simulink model "Target_Control_System"  (R2021b)
settings: Solver=FixedStepDiscrete  StartTime=0.0  StopTime=5  RelTol=1e-3
PreLoadFcn:
  | RTWConfigurationCB('preloadfcn', bdroot);
PostLoadFcn:
  | load('configuration/data_struct.mat');
  | load('configuration/fluxMaps_propMotor.mat');
  | load('configuration/parameterInit_PROP.mat');
  | load('configuration/parameterInit_PUMP.mat');
  | load('configuration/parameterInit_PITCH.mat');
  | load('configuration/parameterInit_TILT.mat');
  | %load('configuration/base_workspace_signal_definition.mat');
  | %load('resolvedatastores_to_baseworkspace_for_faster_simulation.mat');
model workspace (MAT data in the model file):
  SIMULATION_OPTIONS : Simulink.Parameter (value not decoded)
  TARGET_CODE_GEN : Simulink.Parameter (value not decoded)
  TCS_SAMPLE_FREQ_HZ : Simulink.Parameter (value not decoded)
symbols that are objects in the model workspace (value not decoded): TARGET_CODE_GEN, TCS_SAMPLE_FREQ_HZ
undefined symbols (not defined in the file): A_DQ_REF_LPF_INIT__PITCH, A_DQ_REF_LPF_INIT__PROP, A_DQ_REF_LPF_INIT__PUMP, A_DQ_REF_LPF_INIT__TILT, A_OBSERVER_CONFIDENCE_INIT__PITCH, A_OBSERVER_CONFIDENCE_INIT__PROP, A_OBSERVER_CONFIDENCE_INIT__PUMP, A_OBSERVER_CONFIDENCE_INIT__TILT, ACTUATOR_MAX_ANGLE_TRIP__PITCH, ACTUATOR_MIN_ANGLE_TRIP__PITCH, ACTUATOR_POS_SENSOR_INV_DIRECTION__PITCH, ACTUATOR_POS_SENSOR_INV_DIRECTION__TILT, ACTUATOR_POS_SENSOR_OFFSET__PITCH, ACTUATOR_POS_SENSOR_OFFSET__TILT, ADC_scaler1_baseaddr_TILT, ADC_SCALER_FLOAT_TO_FIXPOINT_EXPANSION, ANGLE_ELEC_FROM_SENSOR_OFFSET_INIT__PITCH, ANGLE_ELEC_FROM_SENSOR_OFFSET_INIT__PROP, ANGLE_ELEC_FROM_SENSOR_OFFSET_INIT__PUMP, ANGLE_ELEC_FROM_SENSOR_OFFSET_INIT__TILT, AUTO_CLEAR_FAULTS_ENABLED__PITCH, AUTO_CLEAR_FAULTS_ENABLED__PROP, AUTO_CLEAR_FAULTS_ENABLED__PUMP, AUTO_CLEAR_FAULTS_ENABLED__TILT, AUTO_CLEAR_FAULTS_WAIT_TICKS__PITCH, AUTO_CLEAR_FAULTS_WAIT_TICKS__PROP, AUTO_CLEAR_FAULTS_WAIT_TICKS__PUMP, AUTO_CLEAR_FAULTS_WAIT_TICKS__TILT, AUTO_I_ZERO_IDLE_TICKS__PITCH, AUTO_I_ZERO_IDLE_TICKS__PROP, AUTO_I_ZERO_IDLE_TICKS__PUMP, AUTO_I_ZERO_IDLE_TICKS__TILT, AUTO_I_ZERO_OFFSET_IDC_THRESHOLD__PITCH, AUTO_I_ZERO_OFFSET_IDC_THRESHOLD__PROP, AUTO_I_ZERO_OFFSET_IDC_THRESHOLD__PUMP, AUTO_I_ZERO_OFFSET_IDC_THRESHOLD__TILT, AUTO_I_ZERO_OFFSET_IPH_THRESHOLD__PITCH, AUTO_I_ZERO_OFFSET_IPH_THRESHOLD__PROP, AUTO_I_ZERO_OFFSET_IPH_THRESHOLD__PUMP, AUTO_I_ZERO_OFFSET_IPH_THRESHOLD__TILT, AUTO_SENSORLESS_SWITCHOVER_DISABLE_OMEGA, AUTO_SENSORLESS_SWITCHOVER_ENABLE_OMEGA, AUTO_SENSORLESS_SWITCHOVER_MIN_CONFIDENCE, AUXILIARY_PROTECTION_UNIT_BASEADDR__TILT, blanking_max_error_omega_INIT_PITCH, blanking_max_error_omega_INIT_TILT, blanking_max_error_position_INIT_PITCH, blanking_max_error_position_INIT_TILT, BRUTE_START_I_Q_REF_RAMP_SPEED__PITCH, BRUTE_START_I_Q_REF_RAMP_SPEED__PROP, BRUTE_START_I_Q_REF_RAMP_SPEED__PUMP, BRUTE_START_I_Q_REF_RAMP_SPEED__TILT, CONTROL_LOOP_DT_INIT__PITCH, CONTROL_LOOP_DT_INIT__PROP, CONTROL_LOOP_DT_INIT__PUMP, CONTROL_LOOP_DT_INIT__TILT, CORRECTION_FILTER_SCALE__PITCH, CORRECTION_FILTER_SCALE__PROP, CORRECTION_FILTER_SCALE__PUMP, CORRECTION_FILTER_SCALE__TILT ... (+458)
libraries: simulink x178, Reusables_Lib x24
(part 39 of 47)

== system Target_Control_System/Target_Control_System/MainLoop/tiltMotor_mainLoop/mainTask_tilt/motorTaskMainFastStep(&oTilt)/Mechanical System - Tilt/processSensors(&oPitch)/Output (actuator) side sensor ==
  note: // Ensure the angle is within -pi/2 to pi*1.5 (no loop needed, assuming 'fActuatorSensorOffsetAngle_' is within -pi to pi)
      |    // The reason for this 'skewed' wrap around angle: the tilt sensor on the linkage style tilts moves between 0 and 200 deg,
      |    // so it'd be mighty convenient if it doesn't wrap around at 180 deg. The flaps have a similar situation.
      |    // For pivot style tilt and VP, the sensor moves between -15 deg and 100 deg at most, so the the shifted wrapping point is a non-issue.
  Add1 : Sum
  Add2 : Sum
  Constant20 : Constant  Value=pi  OutDataTypeStr=single  SampleTime=-1
  Constant21 : Constant  Value=2*pi  OutDataTypeStr=single  SampleTime=-1
  Constant23 : Constant  Value=pi  OutDataTypeStr=single  SampleTime=-1
  Constant24 : Constant  Value=2*pi  OutDataTypeStr=single  SampleTime=-1
  Data Store Read1 : DataStoreRead  DataStoreName=oTilt  DataStoreElements=oTilt.oMot_.oState_.oPosSensor_.iActuatorSensorInverseDirection_  IndexOptions=Index vector (dialog)  Indices=1  OutputSizes=1
  Data Store Read2 : DataStoreRead  DataStoreName=oTilt  DataStoreElements=oTilt.oMot_.oIn_.oAdcData_.fOutputEncoderFloat_  IndexOptions=Index vector (dialog)  Indices=1  OutputSizes=1
  Data Store Read3 : DataStoreRead  DataStoreName=oTilt  DataStoreElements=oTilt.oMot_.oState_.oPosSensor_.fActuatorSensorOffsetAngle_  IndexOptions=Index vector (dialog)  Indices=1  OutputSizes=1
  Data Store Write1 : DataStoreWrite  DataStoreName=oTilt  DataStoreElements=oTilt.oMot_.oState_.oPosSensor_.fActuatorAngleFromSensor_  IndexOptions=Index vector (dialog)  Indices=1  OutputSizes=1
  Subtract3 : Sum  Inputs=+-
  Subtract4 : Sum  Inputs=+-
  Subtract8 : Sum  Inputs=-+
  Switch13 : Switch  Criteria=u2 > Threshold
  Switch15 : Switch  Criteria=u2 > Threshold  Threshold=1.5*pi
  Switch5 : Switch  Threshold=-pi/2.0
  wires:
  Subtract8/1 -> Switch15/1
  Constant24/1 -> Add2/2
  Add1/1 -> Subtract8/2, Add2/1, Switch5/2, Switch5/1, Switch15/2
  Data Store Read3/1 -> Add1/1
  Add2/1 -> Switch5/3
  Subtract4/1 -> Switch13/3
  Data Store Read2/1 -> Subtract3/2, Subtract4/1
  Data Store Read1/1 -> Switch13/2
  Subtract3/1 -> Switch13/1
  Constant21/1 -> Subtract8/1
  Switch5/1 -> Switch15/3
  Constant23/1 -> Subtract3/1
  Constant20/1 -> Subtract4/2
  Switch15/1 -> Data Store Write1/1
  Switch13/1 -> Add1/2

== system Target_Control_System/Target_Control_System/MainLoop/tiltMotor_mainLoop/mainTask_tilt/motorTaskMainFastStep(&oTilt)/Motor Acceleration - Tilt/First filter stage/softwareIirFilterStep() ==
  newInput : Inport
  afConstantsB0 : Inport  Port=2
  afConstantsB1 : Inport  Port=3
  afConstantsB2 : Inport  Port=4
  afConstantsA0 : Inport  Port=5
  afConstantsA1 : Inport  Port=6
  afConstantsA2 : Inport  Port=7
  afPreviousInputs0 : Inport  Port=8
  afPreviousInputs1 : Inport  Port=9
  afPreviousOutputs0 : Inport  Port=10
  afPreviousOutputs1 : Inport  Port=11
  Add : Sum  Inputs=+++--
  Constant : Constant  Value=0  OutDataTypeStr=single  SampleTime=-1
  Constant1 : Constant  Value=0  OutDataTypeStr=single  SampleTime=-1
  Divide{,1..5} (6 alike) : Product  Inputs=**
  IsInf : RelationalOperator  Operator=isInf  OutDataTypeStr=boolean  RndMeth=Simplest
  IsInf1 : RelationalOperator  Operator=isInf  OutDataTypeStr=boolean  RndMeth=Simplest
  IsNaN : RelationalOperator  Operator=isNaN  OutDataTypeStr=boolean  RndMeth=Simplest
  IsNaN1 : RelationalOperator  Operator=isNaN  OutDataTypeStr=boolean  RndMeth=Simplest
  Switch{,1..3} (4 alike) : Switch  Criteria=u2 > Threshold
  *afPreviousInputs1 : Outport
  *afPreviousInputs0 : Outport  Port=2
  *afPreviousOutputs1 : Outport  Port=3
  *afPreviousOutputs0 : Outport  Port=4
  fFilterOutput : Outport  Port=5
  wires:
  Switch3/1 -> Divide5/1, *afPreviousOutputs0/1
  IsInf1/1 -> Switch3/2
  IsNaN1/1 -> Switch2/2
  Constant1/1 -> Switch2/1, Switch3/1
  Switch2/1 -> IsInf1/1, Switch3/3
  Add/1 -> IsNaN1/1, Switch2/3  "fOutput"
  Switch1/1 -> Divide/1, *afPreviousInputs0/1
  Switch/1 -> IsInf/1, Switch1/3
  IsInf/1 -> Switch1/2
  Constant/1 -> Switch/1, Switch1/1
  IsNaN/1 -> Switch/2
  Divide5/1 -> fFilterOutput/1
  afConstantsA0/1 -> Divide5/2
  afPreviousOutputs1/1 -> Divide4/1
  afConstantsA2/1 -> Divide4/2
  afPreviousOutputs0/1 -> Divide3/1, *afPreviousOutputs1/1
  afConstantsA1/1 -> Divide3/2
  afPreviousInputs1/1 -> Divide2/1
  afConstantsB2/1 -> Divide2/2
  Divide4/1 -> Add/5
  Divide3/1 -> Add/4
  Divide/1 -> Add/1
  Divide1/1 -> Add/2
  Divide2/1 -> Add/3
  afPreviousInputs0/1 -> Divide1/1, *afPreviousInputs1/1
  afConstantsB1/1 -> Divide1/2
  newInput/1 -> IsNaN/1, Switch/3
  afConstantsB0/1 -> Divide/2

== system Target_Control_System/Target_Control_System/MainLoop/tiltMotor_mainLoop/mainTask_tilt/motorTaskMainFastStep(&oTilt)/Software Overcurrent Protection - Tilt/checkForHwOvercurrents(&oTilt)/gateDriverStatus ==
  note: 1) Add Subsystem or Model blocks as valid variant choices.
      | 2) You cannot connect blocks at this level. At simulation, connectivity is automatically
      | determined, based on the active variant and port name matching.
  DoNotIncludeCustomCode : Subsystem  TreatAsAtomicUnit=on  VariantControl=TARGET_CODE_GEN == 0
  IncludeCustomCode : Subsystem  TreatAsAtomicUnit=on  VariantControl=(default)

== system Target_Control_System/Target_Control_System/Simulation Controls/Simulation Data Store Initialization/setTiltMotorSpecificParameters()/Enabled Subsystem MotorType/Switch Case Action Subsystem MotorType3/softwareIirFilterInitialize()/computeCoefficientsButter() ==
  fCutoffFrequencyHz : Inport  OutDataTypeStr=single
  dSampleFrequencyHz : Inport  Port=2  OutDataTypeStr=single
  Add : Sum  Inputs=+++  OutDataTypeStr=double
  Add1 : Sum  Inputs=-+
  Add2 : Sum  Inputs=+-+  OutDataTypeStr=double
  Constant : Constant  Value=0.0008  OutDataTypeStr=single
  Constant1 : Constant  Value=0.45  OutDataTypeStr=single
  Constant{5,7,9..10} (4 alike) : Constant
  Constant2 : Constant  Value=pi  OutDataTypeStr=double
  Constant3 : Constant  OutDataTypeStr=double
  Constant4 : Constant  Value=sqrt(2)  OutDataTypeStr=double
  Constant6 : Constant  OutDataTypeStr=double
  Constant8 : Constant  Value=2
  Data Type Conversion : DataTypeConversion  OutDataTypeStr=double
  Divide : Product  Inputs=**  OutDataTypeStr=single
  Divide1 : Product  Inputs=**  OutDataTypeStr=single
  Divide{3,5..6,8,10..11} (6 alike) : Product  Inputs=**  OutDataTypeStr=double
  Divide2 : Product  Inputs=*/  OutDataTypeStr=double
  Divide4 : Product  Inputs=*/  OutDataTypeStr=double
  Divide7 : Product  Inputs=*/  OutDataTypeStr=double
  Divide9 : Product  Inputs=***  OutDataTypeStr=double
  Gain : Gain  Gain=2  OutDataTypeStr=double
  Gain1 : Gain  Gain=-1  OutDataTypeStr=double
  Gain2 : Gain  Gain=-1  OutDataTypeStr=double
  Gain3 : Gain  Gain=-1  OutDataTypeStr=double
  Mux : Mux  Inputs=6
  Saturation Dynamic : simulink/Discontinuities/Saturation Dynamic  OutMin=[]  OutMax=[]  OutDataTypeStr=Inherit: Same as second input  OutDataType=fixdt(1, 16)  OutScaling=2^-10  DoSatur=off
  Tan : Trigonometry  Operator=tan
  dpOutArray : Outport
  fFreq3db : Outport  Port=2
  wires:
  Divide/1 -> Saturation Dynamic/3
  Constant1/1 -> Divide1/1
  dSampleFrequencyHz/1 -> Divide/1, Divide2/2, Divide1/2
  Divide1/1 -> Saturation Dynamic/1
  fCutoffFrequencyHz/1 -> Saturation Dynamic/2  "fCutoffFrequencyHz"
  Constant/1 -> Divide/2
  Divide2/1 -> Divide3/1  "dFf"
  Constant2/1 -> Divide3/2
  Divide3/1 -> Tan/1
  Tan/1 -> Divide4/2
  Constant3/1 -> Divide4/1
  Divide4/1 -> [kdIta]
  Constant4/1 -> [kdQ]
  Mux/1 -> dpOutArray/1
  [kdIta] -> Divide6/2, Divide6/1, Divide5/1
  [kdQ] -> Divide5/2
  Divide6/1 -> Add/1
  Divide5/1 -> Add/2
  Constant5/1 -> Add/3
  Constant6/1 -> Divide7/1
  Add/1 -> Divide7/2
  Divide7/1 -> Divide11/1, Divide9/1, [dB2], Gain/1, [dB0]
  Gain/1 -> [dB1]
  [kdIta] -> Divide10/1, Divide8/2, Divide8/1
  Add1/1 -> Divide9/2
  Constant8/1 -> Divide9/3
  Divide9/1 -> [dA1]
  Divide8/1 -> Add2/1, Add1/2
  Constant7/1 -> Add1/1
  [kdQ] -> Divide10/2
  Divide10/1 -> Add2/2
  Constant9/1 -> Add2/3
  Add2/1 -> Gain1/1
  Gain1/1 -> Divide11/2
  Divide11/1 -> [dA2]
  [dB0] -> Mux/1
  [dB1] -> Mux/2
  [dB2] -> Mux/3
  Gain2/1 -> Mux/5
  [dA1] -> Gain2/1
  Gain3/1 -> Mux/6
  [dA2] -> Gain3/1
  Constant10/1 -> Mux/4
  Data Type Conversion/1 -> Divide2/1
  Saturation Dynamic/1 -> fFreq3db/1, Data Type Conversion/1  "fCutoffFrequencyHz"

== system Target_Control_System/Target_Control_System/Simulation Controls/Simulation Data Store Initialization/setupPwm(&oTilt)/setPwmFrequencyApplication()_tilt/setPwmFrequency()_tilt/softwareIirFilterInitialize()/computeCoefficientsButter() ==
  fCutoffFrequencyHz : Inport  OutDataTypeStr=single
  dSampleFrequencyHz : Inport  Port=2  OutDataTypeStr=single
  Add : Sum  Inputs=+++  OutDataTypeStr=double
  Add1 : Sum  Inputs=-+
  Add2 : Sum  Inputs=+-+  OutDataTypeStr=double
  Constant : Constant  Value=0.0008  OutDataTypeStr=single
  Constant1 : Constant  Value=0.45  OutDataTypeStr=single
  Constant{5,7,9..10} (4 alike) : Constant
  Constant2 : Constant  Value=pi  OutDataTypeStr=double
  Constant3 : Constant  OutDataTypeStr=double
  Constant4 : Constant  Value=sqrt(2)  OutDataTypeStr=double
  Constant6 : Constant  OutDataTypeStr=double
  Constant8 : Constant  Value=2
  Data Type Conversion : DataTypeConversion  OutDataTypeStr=double
  Divide : Product  Inputs=**  OutDataTypeStr=single
  Divide1 : Product  Inputs=**  OutDataTypeStr=single
  Divide{3,5..6,8,10..11} (6 alike) : Product  Inputs=**  OutDataTypeStr=double
  Divide2 : Product  Inputs=*/  OutDataTypeStr=double
  Divide4 : Product  Inputs=*/  OutDataTypeStr=double
  Divide7 : Product  Inputs=*/  OutDataTypeStr=double
  Divide9 : Product  Inputs=***  OutDataTypeStr=double
  Gain : Gain  Gain=2  OutDataTypeStr=double
  Gain1 : Gain  Gain=-1  OutDataTypeStr=double
  Gain2 : Gain  Gain=-1  OutDataTypeStr=double
  Gain3 : Gain  Gain=-1  OutDataTypeStr=double
  Mux : Mux  Inputs=6
  Saturation Dynamic : simulink/Discontinuities/Saturation Dynamic  OutMin=[]  OutMax=[]  OutDataTypeStr=Inherit: Same as second input  OutDataType=fixdt(1, 16)  OutScaling=2^-10  DoSatur=off
  Tan : Trigonometry  Operator=tan
  dpOutArray : Outport
  fFreq3db : Outport  Port=2
  wires:
  Saturation Dynamic/1 -> Data Type Conversion/1, fFreq3db/1  "fCutoffFrequencyHz"
  Data Type Conversion/1 -> Divide2/1
  Constant10/1 -> Mux/4
  [dA2] -> Gain3/1
  Gain3/1 -> Mux/6
  [dA1] -> Gain2/1
  Gain2/1 -> Mux/5
  [dB2] -> Mux/3
  [dB1] -> Mux/2
  [dB0] -> Mux/1
  Divide11/1 -> [dA2]
  Gain1/1 -> Divide11/2
  Add2/1 -> Gain1/1
  Constant9/1 -> Add2/3
  Divide10/1 -> Add2/2
  [kdQ] -> Divide10/2
  Constant7/1 -> Add1/1
  Divide8/1 -> Add1/2, Add2/1
  Divide9/1 -> [dA1]
  Constant8/1 -> Divide9/3
  Add1/1 -> Divide9/2
  [kdIta] -> Divide8/1, Divide8/2, Divide10/1
  Gain/1 -> [dB1]
  Divide7/1 -> [dB0], Gain/1, [dB2], Divide9/1, Divide11/1
  Add/1 -> Divide7/2
  Constant6/1 -> Divide7/1
  Constant5/1 -> Add/3
  Divide5/1 -> Add/2
  Divide6/1 -> Add/1
  [kdQ] -> Divide5/2
  [kdIta] -> Divide5/1, Divide6/1, Divide6/2
  Mux/1 -> dpOutArray/1
  Constant4/1 -> [kdQ]
  Divide4/1 -> [kdIta]
  Constant3/1 -> Divide4/1
  Tan/1 -> Divide4/2
  Divide3/1 -> Tan/1
  Constant2/1 -> Divide3/2
  Divide2/1 -> Divide3/1  "dFf"
  Constant/1 -> Divide/2
  fCutoffFrequencyHz/1 -> Saturation Dynamic/2  "fCutoffFrequencyHz"
  Divide1/1 -> Saturation Dynamic/1
  dSampleFrequencyHz/1 -> Divide1/2, Divide2/2, Divide/1
  Constant1/1 -> Divide1/1
  Divide/1 -> Saturation Dynamic/3

== system Target_Control_System/Target_Control_System/Simulation Controls/Simulation Data Store Initialization/setupPwm(&oTilt)/setPwmFrequencyApplication()_tilt/setPwmFrequency()_tilt/softwareIirFilterInitialize()1/computeCoefficientsButter() ==
  fCutoffFrequencyHz : Inport  OutDataTypeStr=single
  dSampleFrequencyHz : Inport  Port=2  OutDataTypeStr=single
  Add : Sum  Inputs=+++  OutDataTypeStr=double
  Add1 : Sum  Inputs=-+
  Add2 : Sum  Inputs=+-+  OutDataTypeStr=double
  Constant : Constant  Value=0.0008  OutDataTypeStr=single
  Constant1 : Constant  Value=0.45  OutDataTypeStr=single
  Constant{5,7,9..10} (4 alike) : Constant
  Constant2 : Constant  Value=pi  OutDataTypeStr=double
  Constant3 : Constant  OutDataTypeStr=double
  Constant4 : Constant  Value=sqrt(2)  OutDataTypeStr=double
  Constant6 : Constant  OutDataTypeStr=double
  Constant8 : Constant  Value=2
  Data Type Conversion : DataTypeConversion  OutDataTypeStr=double
  Divide : Product  Inputs=**  OutDataTypeStr=single
  Divide1 : Product  Inputs=**  OutDataTypeStr=single
  Divide{3,5..6,8,10..11} (6 alike) : Product  Inputs=**  OutDataTypeStr=double
  Divide2 : Product  Inputs=*/  OutDataTypeStr=double
  Divide4 : Product  Inputs=*/  OutDataTypeStr=double
  Divide7 : Product  Inputs=*/  OutDataTypeStr=double
  Divide9 : Product  Inputs=***  OutDataTypeStr=double
  Gain : Gain  Gain=2  OutDataTypeStr=double
  Gain1 : Gain  Gain=-1  OutDataTypeStr=double
  Gain2 : Gain  Gain=-1  OutDataTypeStr=double
  Gain3 : Gain  Gain=-1  OutDataTypeStr=double
  Mux : Mux  Inputs=6
  Saturation Dynamic : simulink/Discontinuities/Saturation Dynamic  OutMin=[]  OutMax=[]  OutDataTypeStr=Inherit: Same as second input  OutDataType=fixdt(1, 16)  OutScaling=2^-10  DoSatur=off
  Tan : Trigonometry  Operator=tan
  dpOutArray : Outport
  fFreq3db : Outport  Port=2
  wires:
  Saturation Dynamic/1 -> Data Type Conversion/1, fFreq3db/1
  Data Type Conversion/1 -> Divide2/1
  Constant10/1 -> Mux/4
  [dA2] -> Gain3/1
  Gain3/1 -> Mux/6
  [dA1] -> Gain2/1
  Gain2/1 -> Mux/5
  [dB2] -> Mux/3
  [dB1] -> Mux/2
  [dB0] -> Mux/1
  Divide11/1 -> [dA2]
  Gain1/1 -> Divide11/2
  Add2/1 -> Gain1/1
  Constant9/1 -> Add2/3
  Divide10/1 -> Add2/2
  [kdQ] -> Divide10/2
  Constant7/1 -> Add1/1
  Divide8/1 -> Add1/2, Add2/1
  Divide9/1 -> [dA1]
  Constant8/1 -> Divide9/3
  Add1/1 -> Divide9/2
  [kdIta] -> Divide8/1, Divide8/2, Divide10/1
  Gain/1 -> [dB1]
  Divide7/1 -> [dB0], Gain/1, [dB2], Divide9/1, Divide11/1
  Add/1 -> Divide7/2
  Constant6/1 -> Divide7/1
  Constant5/1 -> Add/3
  Divide5/1 -> Add/2
  Divide6/1 -> Add/1
  [kdQ] -> Divide5/2
  [kdIta] -> Divide5/1, Divide6/1, Divide6/2
  Mux/1 -> dpOutArray/1
  Constant4/1 -> [kdQ]
  Divide4/1 -> [kdIta]
  Constant3/1 -> Divide4/1
  Tan/1 -> Divide4/2
  Divide3/1 -> Tan/1
  Constant2/1 -> Divide3/2
  Divide2/1 -> Divide3/1  "dFf"
  Constant/1 -> Divide/2
  fCutoffFrequencyHz/1 -> Saturation Dynamic/2  "fCutoffFrequencyHz"
  Divide1/1 -> Saturation Dynamic/1
  dSampleFrequencyHz/1 -> Divide1/2, Divide2/2, Divide/1
  Constant1/1 -> Divide1/1
  Divide/1 -> Saturation Dynamic/3

== system Target_Control_System/Target_Control_System/Simulation Controls/Simulation Data Store Initialization/setupPwm(&oTilt)/setPwmFrequencyApplication()_tilt/setPwmFrequency()_tilt/updateServoObserver()_tilt/softwareIirFilterInitialize() ==
  fFreq3db : Inport
  fFreqSample : Inport  Port=2  OutDataTypeStr=single
  Constant : Constant  OutDataTypeStr=single
  Constant1 : Constant  Value=0  OutDataTypeStr=single
  Data Store Write : DataStoreWrite  DataStoreName=oTilt  DataStoreElements=oTilt.oMot_.oState_.oPosSensor_.oInputSensorSpeedFilter_.afConstantsA_.h0  IndexOptions=Index vector (dialog)  Indices=1  OutputSizes=1
  Data Store Write1 : DataStoreWrite  DataStoreName=oTilt  DataStoreElements=oTilt.oMot_.oState_.oPosSensor_.oInputSensorSpeedFilter_.afConstantsA_.h1  IndexOptions=Index vector (dialog)  Indices=1  OutputSizes=1
  Data Store Write10 : DataStoreWrite  DataStoreName=oTilt  DataStoreElements=oTilt.oMot_.oState_.oPosSensor_.oInputSensorSpeedFilter_.fFilterOutput_  IndexOptions=Index vector (dialog)  Indices=1  OutputSizes=1
  Data Store Write2 : DataStoreWrite  DataStoreName=oTilt  DataStoreElements=oTilt.oMot_.oState_.oPosSensor_.oInputSensorSpeedFilter_.afConstantsA_.h2  IndexOptions=Index vector (dialog)  Indices=1  OutputSizes=1
  Data Store Write3 : DataStoreWrite  DataStoreName=oTilt  DataStoreElements=oTilt.oMot_.oState_.oPosSensor_.oInputSensorSpeedFilter_.afConstantsB_.h2  IndexOptions=Index vector (dialog)  Indices=1  OutputSizes=1
  Data Store Write4 : DataStoreWrite  DataStoreName=oTilt  DataStoreElements=oTilt.oMot_.oState_.oPosSensor_.oInputSensorSpeedFilter_.afConstantsB_.h1  IndexOptions=Index vector (dialog)  Indices=1  OutputSizes=1
  Data Store Write5 : DataStoreWrite  DataStoreName=oTilt  DataStoreElements=oTilt.oMot_.oState_.oPosSensor_.oInputSensorSpeedFilter_.afConstantsB_.h0  IndexOptions=Index vector (dialog)  Indices=1  OutputSizes=1
  Data Store Write6 : DataStoreWrite  DataStoreName=oTilt  DataStoreElements=oTilt.oMot_.oState_.oPosSensor_.oInputSensorSpeedFilter_.afPreviousInputs_.h0  IndexOptions=Index vector (dialog)  Indices=1  OutputSizes=1
  Data Store Write7 : DataStoreWrite  DataStoreName=oTilt  DataStoreElements=oTilt.oMot_.oState_.oPosSensor_.oInputSensorSpeedFilter_.afPreviousInputs_.h1  IndexOptions=Index vector (dialog)  Indices=1  OutputSizes=1
  Data Store Write8 : DataStoreWrite  DataStoreName=oTilt  DataStoreElements=oTilt.oMot_.oState_.oPosSensor_.oInputSensorSpeedFilter_.afPreviousOutputs_.h0  IndexOptions=Index vector (dialog)  Indices=1  OutputSizes=1
  Data Store Write9 : DataStoreWrite  DataStoreName=oTilt  DataStoreElements=oTilt.oMot_.oState_.oPosSensor_.oInputSensorSpeedFilter_.afPreviousOutputs_.h1  IndexOptions=Index vector (dialog)  Indices=1  OutputSizes=1
  Data Type Conversion{,1..4} (5 alike) : DataTypeConversion  OutDataTypeStr=single
  Demux : Demux  Outputs=6
  Divide : Product  Inputs=*/  OutDataTypeStr=single
  computeCoefficientsButter() : Subsystem
  fActualFrequencyHz : Outport
  wires:
  fFreqSample/1 -> computeCoefficientsButter()/2(dSampleFrequencyHz)
  Data Type Conversion4/1 -> Data Store Write2/1
  Data Type Conversion3/1 -> Data Store Write1/1
  Data Type Conversion2/1 -> Data Store Write3/1
  Data Type Conversion/1 -> Data Store Write4/1
  Data Type Conversion1/1 -> Data Store Write5/1
  Constant1/1 -> Data Store Write6/1, Data Store Write7/1, Data Store Write9/1, Data Store Write10/1, Data Store Write8/1
  Demux/1 -> Data Type Conversion1/1
  Demux/2 -> Data Type Conversion/1
  Constant/1 -> Divide/1
  Divide/1 -> Data Store Write/1
  Demux/4 -> Divide/2
  Demux/3 -> Data Type Conversion2/1
  Demux/5 -> Data Type Conversion3/1
  Demux/6 -> Data Type Conversion4/1
  computeCoefficientsButter()/1(dpOutArray) -> Demux/1
  fFreq3db/1 -> computeCoefficientsButter()/1(fCutoffFrequencyHz)
  computeCoefficientsButter()/2(fFreq3db) -> fActualFrequencyHz/1

== system Target_Control_System/Target_Control_System/Simulation Controls/Simulation Data Store Initialization/setupPwm()/setPwmFrequencyApplication()_pitch/setPwmFrequency()_pitch/softwareIirFilterInitialize()/computeCoefficientsButter() ==
  fCutoffFrequencyHz : Inport  OutDataTypeStr=single
  dSampleFrequencyHz : Inport  Port=2  OutDataTypeStr=single
  Add : Sum  Inputs=+++  OutDataTypeStr=double
  Add1 : Sum  Inputs=-+
  Add2 : Sum  Inputs=+-+  OutDataTypeStr=double
  Constant : Constant  Value=0.0008  OutDataTypeStr=single
  Constant1 : Constant  Value=0.45  OutDataTypeStr=single
  Constant{5,7,9..10} (4 alike) : Constant
  Constant2 : Constant  Value=pi  OutDataTypeStr=double
  Constant3 : Constant  OutDataTypeStr=double
  Constant4 : Constant  Value=sqrt(2)  OutDataTypeStr=double
  Constant6 : Constant  OutDataTypeStr=double
  Constant8 : Constant  Value=2
  Data Type Conversion : DataTypeConversion  OutDataTypeStr=double
  Divide : Product  Inputs=**  OutDataTypeStr=single
  Divide1 : Product  Inputs=**  OutDataTypeStr=single
  Divide{3,5..6,8,10..11} (6 alike) : Product  Inputs=**  OutDataTypeStr=double
  Divide2 : Product  Inputs=*/  OutDataTypeStr=double
  Divide4 : Product  Inputs=*/  OutDataTypeStr=double
  Divide7 : Product  Inputs=*/  OutDataTypeStr=double
  Divide9 : Product  Inputs=***  OutDataTypeStr=double
  Gain : Gain  Gain=2  OutDataTypeStr=double
  Gain1 : Gain  Gain=-1  OutDataTypeStr=double
  Gain2 : Gain  Gain=-1  OutDataTypeStr=double
  Gain3 : Gain  Gain=-1  OutDataTypeStr=double
  Mux : Mux  Inputs=6
  Saturation Dynamic : simulink/Discontinuities/Saturation Dynamic  OutMin=[]  OutMax=[]  OutDataTypeStr=Inherit: Same as second input  OutDataType=fixdt(1, 16)  OutScaling=2^-10  DoSatur=off
  Tan : Trigonometry  Operator=tan
  dpOutArray : Outport
  fFreq3db : Outport  Port=2
  wires:
  Saturation Dynamic/1 -> Data Type Conversion/1, fFreq3db/1  "fCutoffFrequencyHz"
  Data Type Conversion/1 -> Divide2/1
  Constant10/1 -> Mux/4
  [dA2] -> Gain3/1
  Gain3/1 -> Mux/6
  [dA1] -> Gain2/1
  Gain2/1 -> Mux/5
  [dB2] -> Mux/3
  [dB1] -> Mux/2
  [dB0] -> Mux/1
  Divide11/1 -> [dA2]
  Gain1/1 -> Divide11/2
  Add2/1 -> Gain1/1
  Constant9/1 -> Add2/3
  Divide10/1 -> Add2/2
  [kdQ] -> Divide10/2
  Constant7/1 -> Add1/1
  Divide8/1 -> Add1/2, Add2/1
  Divide9/1 -> [dA1]
  Constant8/1 -> Divide9/3
  Add1/1 -> Divide9/2
  [kdIta] -> Divide8/1, Divide8/2, Divide10/1
  Gain/1 -> [dB1]
  Divide7/1 -> [dB0], Gain/1, [dB2], Divide9/1, Divide11/1
  Add/1 -> Divide7/2
  Constant6/1 -> Divide7/1
  Constant5/1 -> Add/3
  Divide5/1 -> Add/2
  Divide6/1 -> Add/1
  [kdQ] -> Divide5/2
  [kdIta] -> Divide5/1, Divide6/1, Divide6/2
  Mux/1 -> dpOutArray/1
  Constant4/1 -> [kdQ]
  Divide4/1 -> [kdIta]
  Constant3/1 -> Divide4/1
  Tan/1 -> Divide4/2
  Divide3/1 -> Tan/1
  Constant2/1 -> Divide3/2
  Divide2/1 -> Divide3/1  "dFf"
  Constant/1 -> Divide/2
  fCutoffFrequencyHz/1 -> Saturation Dynamic/2  "fCutoffFrequencyHz"
  Divide1/1 -> Saturation Dynamic/1
  dSampleFrequencyHz/1 -> Divide1/2, Divide2/2, Divide/1
  Constant1/1 -> Divide1/1
  Divide/1 -> Saturation Dynamic/3

== system Target_Control_System/Target_Control_System/Simulation Controls/Simulation Data Store Initialization/setupPwm()/setPwmFrequencyApplication()_pitch/setPwmFrequency()_pitch/softwareIirFilterInitialize()1/computeCoefficientsButter() ==
  fCutoffFrequencyHz : Inport  OutDataTypeStr=single
  dSampleFrequencyHz : Inport  Port=2  OutDataTypeStr=single
  Add : Sum  Inputs=+++  OutDataTypeStr=double
  Add1 : Sum  Inputs=-+
  Add2 : Sum  Inputs=+-+  OutDataTypeStr=double
  Constant : Constant  Value=0.0008  OutDataTypeStr=single  SampleTime=-1
  Constant1 : Constant  Value=0.45  OutDataTypeStr=single  SampleTime=-1
  Constant{5,7,9..10} (4 alike) : Constant  SampleTime=-1
  Constant2 : Constant  Value=pi  OutDataTypeStr=double  SampleTime=-1
  Constant3 : Constant  OutDataTypeStr=double  SampleTime=-1
  Constant4 : Constant  Value=sqrt(2)  OutDataTypeStr=double  SampleTime=-1
  Constant6 : Constant  OutDataTypeStr=double  SampleTime=-1
  Constant8 : Constant  Value=2  SampleTime=-1
  Data Type Conversion : DataTypeConversion  OutDataTypeStr=double
  Divide : Product  Inputs=**  OutDataTypeStr=single
  Divide1 : Product  Inputs=**  OutDataTypeStr=single
  Divide{3,5..6,8,10..11} (6 alike) : Product  Inputs=**  OutDataTypeStr=double
  Divide2 : Product  Inputs=*/  OutDataTypeStr=double
  Divide4 : Product  Inputs=*/  OutDataTypeStr=double
  Divide7 : Product  Inputs=*/  OutDataTypeStr=double
  Divide9 : Product  Inputs=***  OutDataTypeStr=double
  Gain : Gain  Gain=2  OutDataTypeStr=double
  Gain1 : Gain  Gain=-1  OutDataTypeStr=double
  Gain2 : Gain  Gain=-1  OutDataTypeStr=double
  Gain3 : Gain  Gain=-1  OutDataTypeStr=double
  Mux : Mux  Inputs=6
  Saturation Dynamic : simulink/Discontinuities/Saturation Dynamic  OutMin=[]  OutMax=[]  OutDataTypeStr=Inherit: Same as second input  OutDataType=fixdt(1, 16)  OutScaling=2^-10  DoSatur=off
  Tan : Trigonometry  Operator=tan
  dpOutArray : Outport
  fFreq3db : Outport  Port=2
  wires:
  Saturation Dynamic/1 -> Data Type Conversion/1, fFreq3db/1
  Data Type Conversion/1 -> Divide2/1
  Constant10/1 -> Mux/4
  [dA2] -> Gain3/1
  Gain3/1 -> Mux/6
  [dA1] -> Gain2/1
  Gain2/1 -> Mux/5
  [dB2] -> Mux/3
  [dB1] -> Mux/2
  [dB0] -> Mux/1
  Divide11/1 -> [dA2]
  Gain1/1 -> Divide11/2
  Add2/1 -> Gain1/1
  Constant9/1 -> Add2/3
  Divide10/1 -> Add2/2
  [kdQ] -> Divide10/2
  Constant7/1 -> Add1/1
  Divide8/1 -> Add1/2, Add2/1
  Divide9/1 -> [dA1]
  Constant8/1 -> Divide9/3
  Add1/1 -> Divide9/2
  [kdIta] -> Divide8/1, Divide8/2, Divide10/1
  Gain/1 -> [dB1]
  Divide7/1 -> [dB0], Gain/1, [dB2], Divide9/1, Divide11/1
  Add/1 -> Divide7/2
  Constant6/1 -> Divide7/1
  Constant5/1 -> Add/3
  Divide5/1 -> Add/2
  Divide6/1 -> Add/1
  [kdQ] -> Divide5/2
  [kdIta] -> Divide5/1, Divide6/1, Divide6/2
  Mux/1 -> dpOutArray/1
  Constant4/1 -> [kdQ]
  Divide4/1 -> [kdIta]
  Constant3/1 -> Divide4/1
  Tan/1 -> Divide4/2
  Divide3/1 -> Tan/1
  Constant2/1 -> Divide3/2
  Divide2/1 -> Divide3/1  "dFf"
  Constant/1 -> Divide/2
  fCutoffFrequencyHz/1 -> Saturation Dynamic/2  "fCutoffFrequencyHz"
  Divide1/1 -> Saturation Dynamic/1
  dSampleFrequencyHz/1 -> Divide1/2, Divide2/2, Divide/1
  Constant1/1 -> Divide1/1
  Divide/1 -> Saturation Dynamic/3

== system Target_Control_System/Target_Control_System/Simulation Controls/Simulation Data Store Initialization/setupPwm()/setPwmFrequencyApplication()_pitch/setPwmFrequency()_pitch/updateServoObserver()_pitch/softwareIirFilterInitialize() ==
  fFreq3db : Inport
  fFreqSample : Inport  Port=2  OutDataTypeStr=single
  Constant : Constant  OutDataTypeStr=single
  Constant1 : Constant  Value=0  OutDataTypeStr=single
  Data Store Write : DataStoreWrite  DataStoreName=oPitch  DataStoreElements=oPitch.oMot_.oState_.oPosSensor_.oInputSensorSpeedFilter_.afConstantsA_.h0  IndexOptions=Index vector (dialog)  Indices=1  OutputSizes=1
  Data Store Write1 : DataStoreWrite  DataStoreName=oPitch  DataStoreElements=oPitch.oMot_.oState_.oPosSensor_.oInputSensorSpeedFilter_.afConstantsA_.h1  IndexOptions=Index vector (dialog)  Indices=1  OutputSizes=1
  Data Store Write10 : DataStoreWrite  DataStoreName=oPitch  DataStoreElements=oPitch.oMot_.oState_.oPosSensor_.oInputSensorSpeedFilter_.fFilterOutput_  IndexOptions=Index vector (dialog)  Indices=1  OutputSizes=1
  Data Store Write2 : DataStoreWrite  DataStoreName=oPitch  DataStoreElements=oPitch.oMot_.oState_.oPosSensor_.oInputSensorSpeedFilter_.afConstantsA_.h2  IndexOptions=Index vector (dialog)  Indices=1  OutputSizes=1
  Data Store Write3 : DataStoreWrite  DataStoreName=oPitch  DataStoreElements=oPitch.oMot_.oState_.oPosSensor_.oInputSensorSpeedFilter_.afConstantsB_.h2  IndexOptions=Index vector (dialog)  Indices=1  OutputSizes=1
  Data Store Write4 : DataStoreWrite  DataStoreName=oPitch  DataStoreElements=oPitch.oMot_.oState_.oPosSensor_.oInputSensorSpeedFilter_.afConstantsB_.h1  IndexOptions=Index vector (dialog)  Indices=1  OutputSizes=1
  Data Store Write5 : DataStoreWrite  DataStoreName=oPitch  DataStoreElements=oPitch.oMot_.oState_.oPosSensor_.oInputSensorSpeedFilter_.afConstantsB_.h0  IndexOptions=Index vector (dialog)  Indices=1  OutputSizes=1
  Data Store Write6 : DataStoreWrite  DataStoreName=oPitch  DataStoreElements=oPitch.oMot_.oState_.oPosSensor_.oInputSensorSpeedFilter_.afPreviousInputs_.h0  IndexOptions=Index vector (dialog)  Indices=1  OutputSizes=1
  Data Store Write7 : DataStoreWrite  DataStoreName=oPitch  DataStoreElements=oPitch.oMot_.oState_.oPosSensor_.oInputSensorSpeedFilter_.afPreviousInputs_.h1  IndexOptions=Index vector (dialog)  Indices=1  OutputSizes=1
  Data Store Write8 : DataStoreWrite  DataStoreName=oPitch  DataStoreElements=oPitch.oMot_.oState_.oPosSensor_.oInputSensorSpeedFilter_.afPreviousOutputs_.h0  IndexOptions=Index vector (dialog)  Indices=1  OutputSizes=1
  Data Store Write9 : DataStoreWrite  DataStoreName=oPitch  DataStoreElements=oPitch.oMot_.oState_.oPosSensor_.oInputSensorSpeedFilter_.afPreviousOutputs_.h1  IndexOptions=Index vector (dialog)  Indices=1  OutputSizes=1
  Data Type Conversion{,1..4} (5 alike) : DataTypeConversion  OutDataTypeStr=single
  Demux : Demux  Outputs=6
  Divide : Product  Inputs=*/  OutDataTypeStr=single
  computeCoefficientsButter() : Subsystem
  fActualFrequencyHz : Outport
  wires:
  fFreqSample/1 -> computeCoefficientsButter()/2(dSampleFrequencyHz)
  Data Type Conversion4/1 -> Data Store Write2/1
  Data Type Conversion3/1 -> Data Store Write1/1
  Data Type Conversion2/1 -> Data Store Write3/1
  Data Type Conversion/1 -> Data Store Write4/1
  Data Type Conversion1/1 -> Data Store Write5/1
  Constant1/1 -> Data Store Write6/1, Data Store Write7/1, Data Store Write9/1, Data Store Write10/1, Data Store Write8/1
  Demux/1 -> Data Type Conversion1/1
  Demux/2 -> Data Type Conversion/1
  Constant/1 -> Divide/1
  Divide/1 -> Data Store Write/1
  Demux/4 -> Divide/2
  Demux/3 -> Data Type Conversion2/1
  Demux/5 -> Data Type Conversion3/1
  Demux/6 -> Data Type Conversion4/1
  computeCoefficientsButter()/1(dpOutArray) -> Demux/1
  fFreq3db/1 -> computeCoefficientsButter()/1(fCutoffFrequencyHz)
  computeCoefficientsButter()/2(fFreq3db) -> fActualFrequencyHz/1

== system Target_Control_System/Target_Control_System/MainLoop/pitchMotor_mainLoop/Decimation gate for 200 Hz Pitch/Function-Call Subsystem/Position control checks/Position control mode/Check AD2S1210/Enabled Subsystem ==
  Enable : EnablePort
  Chart : Stateflow chart  TreatAsAtomicUnit=on

== system Target_Control_System/Target_Control_System/MainLoop/pitchMotor_mainLoop/Decimation gate for 200 Hz Pitch/Function-Call Subsystem/Position control checks/Position control mode/Check fighting controllers/Enabled Subsystem ==
  note: Notes:
      | opStates->fIqRefBeforeRamp_ is the Iq setpoint (from the speed controller when doing closed loop position and speed control)
      | opIn->fIqSetpoint_        is the Iq setpoint from the other inverter's speed controller (assuming the A<->B inverter link is working)
      | If the two Iq setpoints both exceed an absolute threshold, but have an opposite sign, the controllers are 'fighting'.
      | If the controllers are fighting, turn of the slave controller. (Slave being determined by the 'slave_start' property being set.)
  Enable : EnablePort
  Constant : Constant  Value=0  OutDataTypeStr=uint32  SampleTime=-1
  Data Store Read : DataStoreRead  DataStoreName=oPitch  DataStoreElements=oPitch.oMot_.oParam_.uiSlaveRole_  IndexOptions=Index vector (dialog)  Indices=1  OutputSizes=1
  Enabled Subsystem : Subsystem  TreatAsAtomicUnit=on
  GreaterThan : RelationalOperator  Operator=>  OutDataTypeStr=boolean  RndMeth=Simplest
  wires:
  Constant/1 -> GreaterThan/2
  GreaterThan/1 -> Enabled Subsystem/Enable
  Data Store Read/1 -> GreaterThan/1

== system Target_Control_System/Target_Control_System/MainLoop/pitchMotor_mainLoop/Decimation gate for 200 Hz Pitch/Function-Call Subsystem/Position control checks/Position control mode/checkSensorLimits(&oPitch)/Check broken sensor ==
  note: // Check for a dead or failed input sensor. ('Dead' is not reading; 'failed' is reading, but the sensor tells us it is broken)
  function : TriggerPort  TriggerType=function-call  VariantControl=Variant
  All other sensor types : Subsystem  TreatAsAtomicUnit=on
  Data Store Read : DataStoreRead  DataStoreName=oPitch  DataStoreElements=oPitch.oMot_.oState_.oPosSensor_.eInputPositionSensorType_  IndexOptions=Index vector (dialog)  Indices=1  OutputSizes=1
  Enumerated Constant : simulink/Sources/Enumerated Constant  OutDataTypeStr=Enum: EPositionSensor_t  Value=EPositionSensor_t.eResolver  SampleTime=-1
  Equal : RelationalOperator  Operator===  OutDataTypeStr=boolean  RndMeth=Simplest
  NOT : Logic  Operator=NOT  IconShape=distinctive  AllPortsSameDT=off  OutDataTypeStr=boolean
  Resolver : Subsystem  TreatAsAtomicUnit=on
  wires:
  NOT/1 -> All other sensor types/Enable
  Equal/1 -> Resolver/Enable, NOT/1
  Enumerated Constant/1 -> Equal/2
  Data Store Read/1 -> Equal/1

== system Target_Control_System/Target_Control_System/MainLoop/pitchMotor_mainLoop/Decimation gate for 200 Hz Pitch/Function-Call Subsystem/Position control checks/Position control mode/checkSensorLimits(&oPitch)/Check delta input-output ==
  function : TriggerPort  TriggerType=function-call  VariantControl=Variant
  Constant : Constant  Value=0  OutDataTypeStr=int32  SampleTime=-1
  Data Store Read : DataStoreRead  DataStoreName=oPitch  DataStoreElements=oPitch.oMot_.oState_.oPosSensor_.fInputToOutputSensorMaxDifference_  IndexOptions=Index vector (dialog)  Indices=1  OutputSizes=1
  Enabled Subsystem : Subsystem  TreatAsAtomicUnit=on
  NotEqual : RelationalOperator  Operator=~=  OutDataTypeStr=boolean  RndMeth=Simplest
  wires:
  NotEqual/1 -> Enabled Subsystem/Enable
  Constant/1 -> NotEqual/2
  Data Store Read/1 -> NotEqual/1

== system Target_Control_System/Target_Control_System/MainLoop/pitchMotor_mainLoop/Decimation gate for 200 Hz Pitch/Function-Call Subsystem/Position control checks/Position control mode/checkSensorLimits(&oPitch)/Check for stuck sensor ==
  note: Check for a stuck sensor (a stuck sensor appears to be reading normally and without error codes, but the value doesn't change)
      | (Disabled when iAngleElecFromSensorIdenticalValuesTripMax_ == 0)
  function : TriggerPort  TriggerType=function-call  VariantControl=Variant
  AND : Logic  AllPortsSameDT=off  OutDataTypeStr=boolean
  Constant : Constant  Value=0  OutDataTypeStr=int32  SampleTime=-1
  Data Store Read : DataStoreRead  DataStoreName=oPitch  DataStoreElements=oPitch.oMot_.oState_.oPosSensor_.iAngleElecFromSensorNumOfIdenticalValues_  IndexOptions=Index vector (dialog)  Indices=1  OutputSizes=1
  Data Store Read1 : DataStoreRead  DataStoreName=oPitch  DataStoreElements=oPitch.oMot_.oState_.oPosSensor_.iAngleElecFromSensorIdenticalValuesTripMax_  IndexOptions=Index vector (dialog)  Indices=1  OutputSizes=1
  Enabled Subsystem : Subsystem  TreatAsAtomicUnit=on
  GreaterThan : RelationalOperator  Operator=>  OutDataTypeStr=boolean  RndMeth=Simplest
  GreaterThan1 : RelationalOperator  Operator=>  OutDataTypeStr=boolean  RndMeth=Simplest
  wires:
  AND/1 -> Enabled Subsystem/Enable
  GreaterThan/1 -> AND/2
  GreaterThan1/1 -> AND/1
  Data Store Read/1 -> GreaterThan1/1
  Constant/1 -> GreaterThan/2
  Data Store Read1/1 -> GreaterThan/1, GreaterThan1/2

== system Target_Control_System/Target_Control_System/MainLoop/pitchMotor_mainLoop/Decimation gate for 200 Hz Pitch/Function-Call Subsystem/Position control checks/Position control mode/checkSensorLimits(&oPitch)/Check limits ==
  function : TriggerPort  TriggerType=function-call  VariantControl=Variant
  Chart : Stateflow chart  TreatAsAtomicUnit=on

== system Target_Control_System/Target_Control_System/MainLoop/pitchMotor_mainLoop/Decimation gate for 200 Hz Pitch/Function-Call Subsystem/Position control checks/Position control mode/checkSensorLimits(&oPitch)/Read sensor flags ==
  note: // Reading the sensor flags is somewhat slow (they live on the AXI bus); so read them once beforehand, then run the checks.
  function : TriggerPort  TriggerType=function-call  VariantControl=Variant
  Data Store Read : DataStoreRead  DataStoreName=oPitch  DataStoreElements=oPitch.oMot_.oState_.oPosSensor_.eInputPositionSensorType_  IndexOptions=Index vector (dialog)  Indices=1  OutputSizes=1
  Enumerated Constant : simulink/Sources/Enumerated Constant  OutDataTypeStr=Enum: EPositionSensor_t  Value=EPositionSensor_t.eResolver  SampleTime=-1
  Equal : RelationalOperator  Operator===  OutDataTypeStr=boolean  RndMeth=Simplest
  NOT : Logic  Operator=NOT  IconShape=distinctive  AllPortsSameDT=off  OutDataTypeStr=boolean
  nonresolverSensorCodes : Subsystem  TreatAsAtomicUnit=on
  resolverSensorCodes : Subsystem  TreatAsAtomicUnit=on
  wires:
  Data Store Read/1 -> Equal/1
  Enumerated Constant/1 -> Equal/2
  NOT/1 -> nonresolverSensorCodes/Enable
  Equal/1 -> resolverSensorCodes/Enable, NOT/1

== system Target_Control_System/Target_Control_System/MainLoop/pitchMotor_mainLoop/Decimation gate for 5000 Hz Pitch/motorTaskProcessExternalSetpoints(&oPitch)/set_target/Iq_target/Subsystem/Dynamic Current Limiting Prop ==
  Enable : EnablePort
  Data Store Read68 : DataStoreRead  DataStoreName=oPitch  DataStoreElements=oPitch.oMot_.oIn_.fIqSetpoint_  IndexOptions=Index vector (dialog)  Indices=1  OutputSizes=1
  Data Store Read80 : DataStoreRead  DataStoreName=oPitch  DataStoreElements=oPitch.oMot_.oParam_.fIqSetpointMax_  IndexOptions=Index vector (dialog)  Indices=1  OutputSizes=1
  Gain1 : Gain  Gain=-1
  Max1 : MinMax  Function=max  Inputs=2
  Min : MinMax  Inputs=2
  fIqRefBeforeRamp_ : Outport
  wires:
  Min/1 -> Max1/1
  Data Store Read80/1 -> Gain1/1, Min/2
  Gain1/1 -> Max1/2
  Data Store Read68/1 -> Min/1
  Max1/1 -> fIqRefBeforeRamp_/1

== system Target_Control_System/Target_Control_System/MainLoop/pitchMotor_mainLoop/Decimation gate for 5000 Hz Pitch/motorTaskProcessExternalSetpoints(&oPitch)/set_target/position_target/Subsystem/Current Limiting Prop ==
  oRampDataPos_.fSetpoint_ : Inport
  Enable : EnablePort
  Data Store Read1 : DataStoreRead  DataStoreName=oPitch  DataStoreElements=oPitch.oMot_.oParam_.fPositionSetpointMin_  IndexOptions=Index vector (dialog)  Indices=1  OutputSizes=1
  Data Store Read74 : DataStoreRead  DataStoreName=oPitch  DataStoreElements=oPitch.oMot_.oParam_.fPositionSetpointMax_  IndexOptions=Index vector (dialog)  Indices=1  OutputSizes=1
  Data Store Write1 : DataStoreWrite  DataStoreName=oPitch  DataStoreElements=oPitch.oMot_.oState_.oRampDataPos_.fSetpoint_  IndexOptions=Index vector (dialog)  Indices=1  OutputSizes=1
  Saturation Dynamic : simulink/Discontinuities/Saturation Dynamic  OutMin=[]  OutMax=[]  OutDataTypeStr=Inherit: Same as second input  OutDataType=fixdt(1, 16)  OutScaling=2^-10  DoSatur=off
  wires:
  Saturation Dynamic/1 -> Data Store Write1/1
  Data Store Read1/1 -> Saturation Dynamic/3
  Data Store Read74/1 -> Saturation Dynamic/1
  oRampDataPos_.fSetpoint_/1 -> Saturation Dynamic/2

== system Target_Control_System/Target_Control_System/MainLoop/pitchMotor_mainLoop/mainTask_pitch/motorTaskMainFastStep()/Automatic switching to sensorless - Pitch/Automatic switching to sensorless/Switch to sensored /Switch to sensored ==
  note: // 'opIn->fFluxMasterAngle_' is up to this point the sensor less angle
      | // 'opStates->oPosSensor_.fAngleElecFromSensor_' is the angle from the position sensor, and will be the new fFluxMasterAngle_ later on
  Enable : EnablePort
  Angle To +-pi : Subsystem
  Constant : Constant  OutDataTypeStr=int32
  Constant1 : Constant  Value=0  OutDataTypeStr=uint32
  Data Store Read : DataStoreRead  DataStoreName=oPitch  DataStoreElements=oPitch.oMot_.oIn_.fFluxMasterAngle_  IndexOptions=Index vector (dialog)  Indices=1  OutputSizes=1
  Data Store Read1 : DataStoreRead  DataStoreName=oPitch  DataStoreElements=oPitch.oMot_.oState_.oPosSensor_.fAngleElecFromSensor_  IndexOptions=Index vector (dialog)  Indices=1  OutputSizes=1
  Data Store Write : DataStoreWrite  DataStoreName=oPitch  DataStoreElements=oPitch.oMot_.oState_.oRampDataFluxMstrAngFrcd2clsdSmoothn_.fRampOut_  IndexOptions=Index vector (dialog)  Indices=1  OutputSizes=1
  Data Store Write1 : DataStoreWrite  DataStoreName=oPitch  DataStoreElements=oPitch.oIsr_.oParam_.iUseSensorAngle_  IndexOptions=Index vector (dialog)  Indices=1  OutputSizes=1
  Data Store Write2 : DataStoreWrite  DataStoreName=oPitch  DataStoreElements=oPitch.oMot_.oState_.uiSensorlessSwitchoverState_  IndexOptions=Index vector (dialog)  Indices=1  OutputSizes=1
  Sum : Sum  Inputs=|+-
  wires:
  Constant1/1 -> Data Store Write2/1
  Constant/1 -> Data Store Write1/1
  Angle To +-pi/1(Angle Out) -> Data Store Write/1
  Sum/1 -> Angle To +-pi/1(Angle In)
  Data Store Read1/1 -> Sum/2
  Data Store Read/1 -> Sum/1

== system Target_Control_System/Target_Control_System/MainLoop/pitchMotor_mainLoop/mainTask_pitch/motorTaskMainFastStep()/Automatic switching to sensorless - Pitch/Automatic switching to sensorless/Switch to sensorless?/Switch to sensorless ==
  Enable : EnablePort
  Angle To +-pi : Subsystem
  Constant : Constant  Value=0  OutDataTypeStr=int32
  Constant1 : Constant  OutDataTypeStr=uint32
  Data Store Read : DataStoreRead  DataStoreName=oPitch  DataStoreElements=oPitch.oMot_.oIn_.fFluxMasterAngle_  IndexOptions=Index vector (dialog)  Indices=1  OutputSizes=1
  Data Store Read1 : DataStoreRead  DataStoreName=oPitch  DataStoreElements=oPitch.oMot_.oIn_.fFluxMainAngleRaw2_  IndexOptions=Index vector (dialog)  Indices=1  OutputSizes=1
  Data Store Write : DataStoreWrite  DataStoreName=oPitch  DataStoreElements=oPitch.oMot_.oState_.oRampDataFluxMstrAngFrcd2clsdSmoothn_.fRampOut_  IndexOptions=Index vector (dialog)  Indices=1  OutputSizes=1
  Data Store Write1 : DataStoreWrite  DataStoreName=oPitch  DataStoreElements=oPitch.oIsr_.oParam_.iUseSensorAngle_  IndexOptions=Index vector (dialog)  Indices=1  OutputSizes=1
  Data Store Write2 : DataStoreWrite  DataStoreName=oPitch  DataStoreElements=oPitch.oMot_.oState_.uiSensorlessSwitchoverState_  IndexOptions=Index vector (dialog)  Indices=1  OutputSizes=1
  Sum : Sum  Inputs=|+-
  wires:
  Constant1/1 -> Data Store Write2/1
  Constant/1 -> Data Store Write1/1
  Angle To +-pi/1(Angle Out) -> Data Store Write/1
  Sum/1 -> Angle To +-pi/1(Angle In)
  Data Store Read1/1 -> Sum/2
  Data Store Read/1 -> Sum/1

== system Target_Control_System/Target_Control_System/MainLoop/pitchMotor_mainLoop/mainTask_pitch/motorTaskMainFastStep()/Control Loops - Pitch/Speed Controller Pitch/Enabled Subsystem/pid2ControllerStep(oPidDataRpmCtrl)_pitch ==
  fActual : Inport
  fTarget : Inport  Port=2
  fErrorReduction : Inport  Port=3
  fLargeErrorThresholdPositive : Inport  Port=4
  fLargeErrorThresholdNegative : Inport  Port=5
  fBlankingMaxError : Inport  Port=6
  fKi : Inport  Port=7
  ipInhibitTarget : Inport  Port=8
  fLoopDt : Inport  Port=9
  fIntMax : Inport  Port=10
  fIntMin : Inport  Port=11
  fIntegratorLeakFactor : Inport  Port=12
  fKd : Inport  Port=13
  fActualDt : Inport  Port=14
  fDMax : Inport  Port=15
  fDMin : Inport  Port=16
  fKp : Inport  Port=17
  fOutMax : Inport  Port=18
  fOutMin : Inport  Port=19
  fpState : Inport  Port=20
  Abs : Abs
  Abs1 : Abs
  Add : Sum  Inputs=|++
  Add1 : Sum
  Constant : Constant  Value=0  OutDataTypeStr=single  SampleTime=-1
  Constant3 : Constant  Value=0  OutDataTypeStr=single  SampleTime=-1
  Constant4 : Constant  Value=0  OutDataTypeStr=single  SampleTime=-1
  Constant5 : Constant  OutDataTypeStr=single  SampleTime=-1
  Constant6 : Constant  OutDataTypeStr=int32  SampleTime=-1
  Constant7 : Constant  Value=-1  OutDataTypeStr=int32  SampleTime=-1
  Constant8 : Constant  Value=0  OutDataTypeStr=int32  SampleTime=-1
  Divide : Product  Inputs=**
  Divide1 : Product  Inputs=**
  GreaterThan : RelationalOperator  Operator=>  OutDataTypeStr=boolean  RndMeth=Simplest
  GreaterThan1 : RelationalOperator  Operator=<  OutDataTypeStr=boolean  RndMeth=Simplest
  GreaterThan2 : RelationalOperator  OutDataTypeStr=boolean  RndMeth=Simplest
  GreaterThan3 : RelationalOperator  Operator=>  OutDataTypeStr=boolean  RndMeth=Simplest
  GreaterThan4 : RelationalOperator  Operator=>  OutDataTypeStr=boolean  RndMeth=Simplest
  GreaterThan5 : RelationalOperator  Operator=<  OutDataTypeStr=boolean  RndMeth=Simplest
  GreaterThan6 : RelationalOperator  Operator=<  OutDataTypeStr=boolean  RndMeth=Simplest
  OR1 : Logic  AllPortsSameDT=off  OutDataTypeStr=boolean
  OR2 : Logic  AllPortsSameDT=off  OutDataTypeStr=boolean
  OR3 : Logic  Operator=OR  AllPortsSameDT=off  OutDataTypeStr=boolean
  Product{,1..4} (5 alike) : Product
  Saturation : Saturate  UpperLimit=inf  LowerLimit=0
  Saturation Dynamic : simulink/Discontinuities/Saturation Dynamic  OutMin=[]  OutMax=[]  OutDataTypeStr=Inherit: Same as second input  OutDataType=fixdt(1, 16)  OutScaling=2^-10  DoSatur=off
  Saturation Dynamic1 : simulink/Discontinuities/Saturation Dynamic  OutMin=[]  OutMax=[]  OutDataTypeStr=Inherit: Same as second input  OutDataType=fixdt(1, 16)  OutScaling=2^-10  DoSatur=off
  Saturation Dynamic2 : simulink/Discontinuities/Saturation Dynamic  OutMin=[]  OutMax=[]  OutDataTypeStr=Inherit: Same as second input  OutDataType=fixdt(1, 16)  OutScaling=2^-10  DoSatur=off
  Sign : Signum
  Sum : Sum  Inputs=|++
  Sum2 : Sum  Inputs=-+|
  Sum22 : Sum  Inputs=-+|
  Sum4 : Sum  Inputs=+-|
  Switch{1..4} (4 alike) : Switch  Criteria=u2 > Threshold
  Unit Delay2 : UnitDelay  SampleTime=-1  HasFrameUpgradeWarning=on
  iLargeErrorPresent : Outport
  fITerm : Outport  Port=2
  fDTerm : Outport  Port=3
  fPTerm : Outport  Port=4
  fOutput : Outport  Port=5
  *fpState : Outport  Port=6
  wires:
  Switch3/1 -> iLargeErrorPresent/1
  Constant8/1 -> Switch4/3
  Switch4/1 -> Switch3/3
  Constant7/1 -> Switch3/1
  Constant6/1 -> Switch4/1
  GreaterThan/1 -> Switch4/2
  GreaterThan1/1 -> Switch3/2
  Sum/1 -> Saturation Dynamic1/2
  Add1/1 -> Sum/2
  Product4/1 -> fPTerm/1, Sum/1
  fKp/1 -> Product4/1
  Saturation Dynamic2/1 -> fDTerm/1, Add1/1  "fDTerm"
  fDMax/1 -> Saturation Dynamic2/1
  fDMin/1 -> Saturation Dynamic2/3
  Product3/1 -> Saturation Dynamic2/2  "fDTerm"
  fActualDt/1 -> Product3/2
  fKd/1 -> Product3/1
  Unit Delay2/1 -> Product2/1  "*fpState"
  Product2/1 -> fITerm/1, *fpState/1, Add1/2  "*fpState"
  Sum4/1 -> Product2/2
  Constant5/1 -> Sum4/1
  Product1/1 -> Sum4/2
  fIntegratorLeakFactor/1 -> Product1/2
  Saturation Dynamic/1 -> Unit Delay2/1
  Add/1 -> Saturation Dynamic/2  "fpState"
  Switch2/1 -> Product/1  "fErrorForIntegrator"
  Constant4/1 -> Switch2/1
  OR3/1 -> Switch2/2
  OR2/1 -> OR3/2
  OR1/1 -> OR3/1
  GreaterThan6/1 -> OR2/2
  GreaterThan5/1 -> OR2/1
  GreaterThan3/1 -> OR1/2
  GreaterThan4/1 -> OR1/1
  Divide1/1 -> GreaterThan4/1, Switch2/3, GreaterThan5/1  "fErrorForIntegrator"
  Constant3/1 -> GreaterThan3/2, GreaterThan4/2, GreaterThan5/2, GreaterThan6/2
  ipInhibitTarget/1 -> GreaterThan6/1, GreaterThan3/1
  fKi/1 -> Divide1/2
  Switch1/1 -> Divide1/1  "fErrorForIntegrator"
  Constant/1 -> Switch1/3
  GreaterThan2/1 -> Switch1/2
  fBlankingMaxError/1 -> GreaterThan2/2
  Abs1/1 -> GreaterThan2/1
  fLargeErrorThresholdNegative/1 -> GreaterThan1/2
  fLargeErrorThresholdPositive/1 -> GreaterThan/2
  Divide/1 -> GreaterThan/1, GreaterThan1/1, Product4/2, Abs1/1, Switch1/1  "fError"
  Sign/1 -> Divide/2
  Saturation/1 -> Divide/1
  Sum2/1 -> Saturation/1  "fTemp"
  fErrorReduction/1 -> Sum2/1
  Abs/1 -> Sum2/2
  fActual/1 -> Sum22/1
  fOutMax/1 -> Saturation Dynamic1/1
  fpState/1 -> Add/2
  Saturation Dynamic1/1 -> fOutput/1
  fTarget/1 -> Sum22/2
  Product/1 -> Add/1
  Sum22/1 -> Abs/1, Sign/1  "fError"
  fOutMin/1 -> Saturation Dynamic1/3
  fIntMax/1 -> Saturation Dynamic/1
  fLoopDt/1 -> Product/2, Product1/1
  fIntMin/1 -> Saturation Dynamic/3
